simulink model "Pendulum"  (R2013a)
settings: Solver=ode1  SolverMode=SingleTasking  StartTime=0.0  StopTime=inf  FixedStep=0.01  RelTol=1e-3
InitFcn:
  | fuzzycontroller1=readfis('fuzzy1.fis');
  | fuzzycontroller2=readfis('fuzzy2.fis');
  | fuzzypid=readfis('fuzzy3.fis');
libraries: neural x91, fuzblock x9
(part 2 of 2)

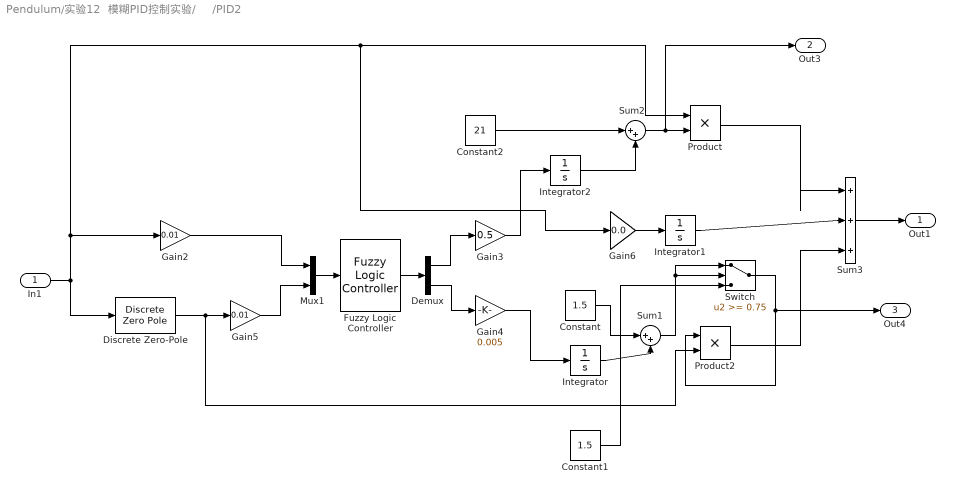
== system Pendulum/实验12  模糊PID控制实验/     /PID2 ==
  In1 : Inport
  Constant : Constant  Value=1.5
  Constant1 : Constant  Value=1.5
  Constant2 : Constant  Value=21
  Demux : Demux  Outputs=2
  Discrete Zero-Pole : DiscreteZeroPole  Poles=[0]  Gain=35  SampleTime=0.01
  Fuzzy Logic Controller : fuzblock/Fuzzy Logic  Controller  fis=fuzzypid
  Gain2 : Gain  Gain=0.01  SaturateOnIntegerOverflow=on  OutDataTypeStr=Inherit: Same as input  ParamDataTypeStr=Inherit: Same as input
  Gain3 : Gain  Gain=0.5  SaturateOnIntegerOverflow=on  OutDataTypeStr=Inherit: Same as input  ParamDataTypeStr=Inherit: Same as input
  Gain4 : Gain  Gain=0.005  SaturateOnIntegerOverflow=on  OutDataTypeStr=Inherit: Same as input  ParamDataTypeStr=Inherit: Same as input
  Gain5 : Gain  Gain=0.01  SaturateOnIntegerOverflow=on  OutDataTypeStr=Inherit: Same as input  ParamDataTypeStr=Inherit: Same as input
  Gain6 : Gain  Gain=0.0  SaturateOnIntegerOverflow=on  OutDataTypeStr=Inherit: Same as input  ParamDataTypeStr=Inherit: Same as input
  Integrator : Integrator
  Integrator1 : Integrator
  Integrator2 : Integrator
  Mux1 : Mux  Inputs=2
  Product : Product  SaturateOnIntegerOverflow=on  OutDataTypeStr=Inherit: Same as first input
  Product2 : Product  SaturateOnIntegerOverflow=on  OutDataTypeStr=Inherit: Same as first input
  Sum1 : Sum  Inputs=|++  SaturateOnIntegerOverflow=on
  Sum2 : Sum  Inputs=|++  SaturateOnIntegerOverflow=on
  Sum3 : Sum  Inputs=|+++  SaturateOnIntegerOverflow=on
  Switch : Switch  Threshold=0.75  SaturateOnIntegerOverflow=on
  Out1 : Outport
  Out3 : Outport  Port=2
  Out4 : Outport  Port=3
  wires:
  Product2/1 -> Sum3/3
  Constant1/1 -> Switch/3
  Sum1/1 -> Switch/2, Switch/1
  Switch/1 -> Out4/1, Product2/1
  Integrator/1 -> Sum1/2
  Sum3/1 -> Out1/1
  Constant/1 -> Sum1/1
  Demux/2 -> Gain4/1
  Gain6/1 -> Integrator1/1
  Product/1 -> Sum3/1
  Gain2/1 -> Mux1/1
  Gain4/1 -> Integrator/1
  Fuzzy Logic Controller/1 -> Demux/1
  Gain5/1 -> Mux1/2
  Demux/1 -> Gain3/1
  Gain3/1 -> Integrator2/1
  Sum2/1 -> Out3/1, Product/2
  Mux1/1 -> Fuzzy Logic Controller/1
  Integrator2/1 -> Sum2/2
  Constant2/1 -> Sum2/1
  Integrator1/1 -> Sum3/2
  Discrete Zero-Pole/1 -> Gain5/1, Product2/2
  In1/1 -> Discrete Zero-Pole/1, Gain2/1, Product/1, Gain6/1

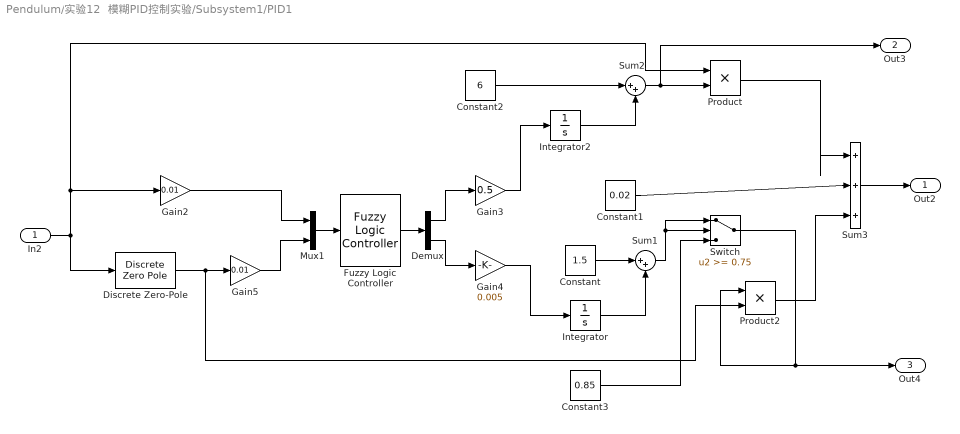
== system Pendulum/实验12  模糊PID控制实验/Subsystem1/PID1 ==
  In2 : Inport
  Constant : Constant  Value=1.5
  Constant1 : Constant  Value=0.02
  Constant2 : Constant  Value=6
  Constant3 : Constant  Value=0.85
  Demux : Demux  Outputs=2
  Discrete Zero-Pole : DiscreteZeroPole  Poles=[0]  Gain=35  SampleTime=0.01
  Fuzzy Logic Controller : fuzblock/Fuzzy Logic  Controller  fis=fuzzypid
  Gain2 : Gain  Gain=0.01  SaturateOnIntegerOverflow=on  OutDataTypeStr=Inherit: Same as input  ParamDataTypeStr=Inherit: Same as input
  Gain3 : Gain  Gain=0.5  SaturateOnIntegerOverflow=on  OutDataTypeStr=Inherit: Same as input  ParamDataTypeStr=Inherit: Same as input
  Gain4 : Gain  Gain=0.005  SaturateOnIntegerOverflow=on  OutDataTypeStr=Inherit: Same as input  ParamDataTypeStr=Inherit: Same as input
  Gain5 : Gain  Gain=0.01  SaturateOnIntegerOverflow=on  OutDataTypeStr=Inherit: Same as input  ParamDataTypeStr=Inherit: Same as input
  Integrator : Integrator
  Integrator2 : Integrator
  Mux1 : Mux  Inputs=2
  Product : Product  SaturateOnIntegerOverflow=on  OutDataTypeStr=Inherit: Same as first input
  Product2 : Product  SaturateOnIntegerOverflow=on  OutDataTypeStr=Inherit: Same as first input
  Sum1 : Sum  Inputs=|++  SaturateOnIntegerOverflow=on
  Sum2 : Sum  Inputs=|++  SaturateOnIntegerOverflow=on
  Sum3 : Sum  Inputs=|+++  SaturateOnIntegerOverflow=on
  Switch : Switch  Threshold=0.75  SaturateOnIntegerOverflow=on
  Out2 : Outport
  Out3 : Outport  Port=2
  Out4 : Outport  Port=3
  wires:
  Sum3/1 -> Out2/1
  Discrete Zero-Pole/1 -> Gain5/1, Product2/2
  Switch/1 -> Out4/1, Product2/1
  Product2/1 -> Sum3/3
  In2/1 -> Discrete Zero-Pole/1, Gain2/1, Product/1
  Constant3/1 -> Switch/3
  Fuzzy Logic Controller/1 -> Demux/1
  Sum2/1 -> Out3/1, Product/2
  Gain5/1 -> Mux1/2
  Constant2/1 -> Sum2/1
  Constant/1 -> Sum1/1
  Mux1/1 -> Fuzzy Logic Controller/1
  Constant1/1 -> Sum3/2
  Integrator/1 -> Sum1/2
  Demux/1 -> Gain3/1
  Demux/2 -> Gain4/1
  Product/1 -> Sum3/1
  Sum1/1 -> Switch/2, Switch/1
  Gain3/1 -> Integrator2/1
  Gain2/1 -> Mux1/1
  Integrator2/1 -> Sum2/2
  Gain4/1 -> Integrator/1

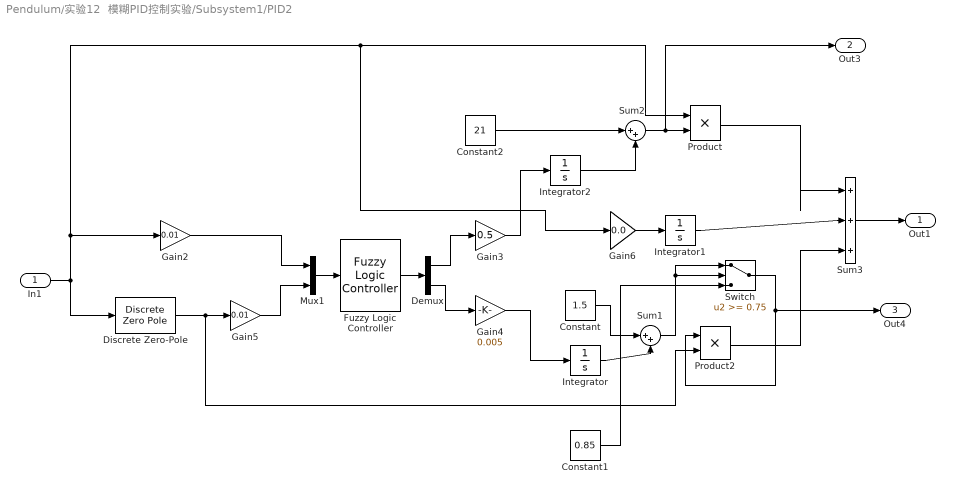
== system Pendulum/实验12  模糊PID控制实验/Subsystem1/PID2 ==
  In1 : Inport
  Constant : Constant  Value=1.5
  Constant1 : Constant  Value=0.85
  Constant2 : Constant  Value=21
  Demux : Demux  Outputs=2
  Discrete Zero-Pole : DiscreteZeroPole  Poles=[0]  Gain=35  SampleTime=0.01
  Fuzzy Logic Controller : fuzblock/Fuzzy Logic  Controller  fis=fuzzypid
  Gain2 : Gain  Gain=0.01  SaturateOnIntegerOverflow=on  OutDataTypeStr=Inherit: Same as input  ParamDataTypeStr=Inherit: Same as input
  Gain3 : Gain  Gain=0.5  SaturateOnIntegerOverflow=on  OutDataTypeStr=Inherit: Same as input  ParamDataTypeStr=Inherit: Same as input
  Gain4 : Gain  Gain=0.005  SaturateOnIntegerOverflow=on  OutDataTypeStr=Inherit: Same as input  ParamDataTypeStr=Inherit: Same as input
  Gain5 : Gain  Gain=0.01  SaturateOnIntegerOverflow=on  OutDataTypeStr=Inherit: Same as input  ParamDataTypeStr=Inherit: Same as input
  Gain6 : Gain  Gain=0.0  SaturateOnIntegerOverflow=on  OutDataTypeStr=Inherit: Same as input  ParamDataTypeStr=Inherit: Same as input
  Integrator : Integrator
  Integrator1 : Integrator
  Integrator2 : Integrator
  Mux1 : Mux  Inputs=2
  Product : Product  SaturateOnIntegerOverflow=on  OutDataTypeStr=Inherit: Same as first input
  Product2 : Product  SaturateOnIntegerOverflow=on  OutDataTypeStr=Inherit: Same as first input
  Sum1 : Sum  Inputs=|++  SaturateOnIntegerOverflow=on
  Sum2 : Sum  Inputs=|++  SaturateOnIntegerOverflow=on
  Sum3 : Sum  Inputs=|+++  SaturateOnIntegerOverflow=on
  Switch : Switch  Threshold=0.75  SaturateOnIntegerOverflow=on
  Out1 : Outport
  Out3 : Outport  Port=2
  Out4 : Outport  Port=3
  wires:
  Product2/1 -> Sum3/3
  Constant1/1 -> Switch/3
  Sum1/1 -> Switch/2, Switch/1
  Switch/1 -> Out4/1, Product2/1
  Integrator/1 -> Sum1/2
  Sum3/1 -> Out1/1
  Constant/1 -> Sum1/1
  Demux/2 -> Gain4/1
  Gain6/1 -> Integrator1/1
  Product/1 -> Sum3/1
  Gain2/1 -> Mux1/1
  Gain4/1 -> Integrator/1
  Fuzzy Logic Controller/1 -> Demux/1
  Gain5/1 -> Mux1/2
  Demux/1 -> Gain3/1
  Gain3/1 -> Integrator2/1
  Sum2/1 -> Out3/1, Product/2
  Mux1/1 -> Fuzzy Logic Controller/1
  Integrator2/1 -> Sum2/2
  Constant2/1 -> Sum2/1
  Integrator1/1 -> Sum3/2
  Discrete Zero-Pole/1 -> Gain5/1, Product2/2
  In1/1 -> Discrete Zero-Pole/1, Gain2/1, Product/1, Gain6/1

== system Pendulum/实验13  神经网络控制实验/神经网络控制器/BP Neural Network ==
  note: 隐层
  note: 输出层
  "p{1}" : Inport  PortDimensions=4
  Layer 1 : Subsystem
  Layer 2 : Subsystem
  "y{1}" : Outport  InitialOutput=0
  wires:
  "p{1}"/1 -> Layer 1/1("p{1}")
  Layer 1/1("a{1}") -> [feedback1]
  [feedback1] -> Layer 2/1("a{1} ")
  Layer 2/1("a{2}") -> "y{1}"/1

== system Pendulum/实验13  神经网络控制实验/神经网络控制器/RBF Neural Network ==
  note: 隐层
  note: 输出层
  "p{1}" : Inport  PortDimensions=4
  Layer 1 : Subsystem
  Layer 2 : Subsystem
  "y{1}" : Outport  InitialOutput=0
  wires:
  "p{1}"/1 -> Layer 1/1("p{1}")
  Layer 1/1("a{1}") -> [feedback1]
  [feedback1] -> Layer 2/1("a{1} ")
  Layer 2/1("a{2}") -> "y{1}"/1

== system Pendulum/实验4  PID控制实验/只对摆杆角度施加控制/PID1 ==
  In1 : Inport
  Discrete Zero-Pole : DiscreteZeroPole  Poles=[0]  Gain=100  SampleTime=0.01
  Gain : Gain  Gain=Kp
  Gain1 : Gain  Gain=Ki
  Gain2 : Gain  Gain=Kd
  Integrator : Integrator  LimitOutput=on  UpperSaturationLimit=0.01  LowerSaturationLimit=-0.01
  Sum : Sum  Inputs=|+++
  Out1 : Outport
  wires:
  Discrete Zero-Pole/1 -> Sum/3
  Gain1/1 -> Integrator/1
  Gain2/1 -> Discrete Zero-Pole/1
  Integrator/1 -> Sum/2
  Gain/1 -> Sum/1
  Sum/1 -> Out1/1
  In1/1 -> Gain2/1, Gain/1, Gain1/1

== system Pendulum/实验4  PID控制实验/对摆杆角度和小车 位置同时施加控制/PID2 ==
  In1 : Inport
  Discrete Zero-Pole : DiscreteZeroPole  Poles=[0]  Gain=100  SampleTime=0.01
  Gain : Gain  Gain=Kp
  Gain1 : Gain  Gain=Ki
  Gain2 : Gain  Gain=Kd
  Integrator : Integrator  LimitOutput=on  UpperSaturationLimit=0.01  LowerSaturationLimit=-0.01
  Sum : Sum  Inputs=|+++
  Out1 : Outport
  wires:
  Discrete Zero-Pole/1 -> Sum/3
  Gain1/1 -> Integrator/1
  Gain2/1 -> Discrete Zero-Pole/1
  Integrator/1 -> Sum/2
  Gain/1 -> Sum/1
  Sum/1 -> Out1/1
  In1/1 -> Gain2/1, Gain/1, Gain1/1

== system Pendulum/实验4  PID控制实验/对摆杆角度和小车 位置同时施加控制/PID3 ==
  In1 : Inport
  Discrete Zero-Pole : DiscreteZeroPole  Poles=[0]  Gain=100  SampleTime=0.01
  Gain : Gain  Gain=Kp
  Gain1 : Gain  Gain=Ki
  Gain2 : Gain  Gain=Kd
  Integrator : Integrator  LimitOutput=on  UpperSaturationLimit=0.01  LowerSaturationLimit=-0.01
  Sum : Sum  Inputs=|+++
  Out1 : Outport
  wires:
  Discrete Zero-Pole/1 -> Sum/3
  Gain1/1 -> Integrator/1
  Gain2/1 -> Discrete Zero-Pole/1
  Integrator/1 -> Sum/2
  Gain/1 -> Sum/1
  Sum/1 -> Out1/1
  In1/1 -> Gain2/1, Gain/1, Gain1/1

== system Pendulum/实验13  神经网络控制实验/神经网络控制器/BP Neural Network/Layer 1 ==
  "p{1}" : Inport  PortDimensions=4
  Delays 1 : Subsystem
      mask Display: disp('TDL')
  "IW{1,1}" : Subsystem
      mask Display: disp('weight')
  "b{1}" : Constant  Value=[-2.6149835398352681;2.2357175048992701;-1.8583595574267076;1.2412188382088436;-0.71456466032423327;0.016058742464604113;-0.094308202124535473;-0.78098051834080862;1.0581145977002466;-1.9595241811893389;2.1672431536686729;2.6034855087406199]
      mask Display: disp('bias')
  netsum : Sum  Inputs=2  SaturateOnIntegerOverflow=on  InputSameDT=on  OutDataTypeStr=Inherit: Same as first input
  tansig : neural/Transfer Functions/tansig
  "a{1}" : Outport  InitialOutput=[0;0;0;0;0;0;0;0;0;0;0;0]
  wires:
  "p{1}"/1 -> Delays 1/1("p{1}")
  Delays 1/1("pd{1,1}") -> "IW{1,1}"/1("pd{1,1}")
  "IW{1,1}"/1("iz{1,1}") -> netsum/1
  "b{1}"/1 -> netsum/2
  netsum/1 -> tansig/1
  tansig/1 -> "a{1}"/1

== system Pendulum/实验13  神经网络控制实验/神经网络控制器/BP Neural Network/Layer 2 ==
  "a{1} " : Inport  PortDimensions=12
  Delays 1 : Subsystem
      mask Display: disp('TDL')
  "LW{2,1}" : Subsystem
      mask Display: disp('weight')
  "b{2}" : Constant  Value=-0.019497373495995372
      mask Display: disp('bias')
  netsum : Sum  Inputs=2  SaturateOnIntegerOverflow=on  InputSameDT=on  OutDataTypeStr=Inherit: Same as first input
  purelin : neural/Transfer Functions/purelin
  "a{2}" : Outport  InitialOutput=0
  wires:
  "a{1} "/1 -> Delays 1/1("p{2}")
  Delays 1/1("pd{2,1}") -> "LW{2,1}"/1("ad{2,1}")
  "LW{2,1}"/1("lz{2,1}") -> netsum/1
  "b{2}"/1 -> netsum/2
  netsum/1 -> purelin/1
  purelin/1 -> "a{2}"/1

== system Pendulum/实验13  神经网络控制实验/神经网络控制器/RBF Neural Network/Layer 1 ==
  "p{1}" : Inport  PortDimensions=4
  Delays 1 : Subsystem
      mask Display: disp('TDL')
  "IW{1,1}" : Subsystem
      mask Display: disp('weight')
  "b{1}" : Constant  Value=[2.7751820371923257;2.7751820371923257;2.7751820371923257;2.7751820371923257;2.7751820371923257;2.7751820371923257;2.7751820371923257;2.7751820371923257;2.7751820371923257;2.7751820371923257;2.7751820371923257;2.7751820371923257;2.7751820371923257;2.7751820371923257;2.7751820371923257;2.7751820371923257;2.7751820371923257;2.7751820371923257;2.7751820371923257;2.7751820371923257;2.7751820371923257;2.7751820371923257;2.7751820371923257;2.7751820371923257;2.7751820371923257;2.7751820371923257;2.7751820371923257;2.7751820371923257;2.7751820371923257;2.7751820371923257;2.7751820371923257;2.7751820371923257;2.7751820371923257;2.7751820371923257;2.7751820371923257;2.7751820371923257;2.7751820371923257;2.7751820371923257;2.7751820371923257;2.7751820371923257;2.7751820371923257;2.7751820371923257;2.7751820371923257;2.7751820371923257;2.7751820371923257;2.7751820371923257;2.7751820371923257;2.7751820371923257;2.7751820371923257;2.7751820371923257;2.7751820371923257;2.7751820371923257;2.7751820371923257;2.7751820371923257;2.7751820371923257;2.7751820371923257;2.7751820371923257;2.7751820371923257;2.7751820371923257;2.7751820371923257;2.7751820371923257;2.7751820371923257;2.7751820371923257;2.7751820371923257;2.7751820371923257;2.7751820371923257;2.7751820371923257;2.7751820371923257;2.7751820371923257;2.7751820371923257;2.7751820371923257;2.7751820371923257;2.7751820371923257]
      mask Display: disp('bias')
  netprod : Product  SaturateOnIntegerOverflow=on  InputSameDT=on  OutDataTypeStr=Inherit: Same as first input
  radbas : neural/Transfer Functions/radbas
  "a{1}" : Outport  InitialOutput=[0;0;0;0;0;0;0;0;0;0;0;0;0;0;0;0;0;0;0;0;0;0;0;0;0;0;0;0;0;0;0;0;0;0;0;0;0;0;0;0;0;0;0;0;0;0;0;0;0;0;0;0;0;0;0;0;0;0;0;0;0;0;0;0;0;0;0;0;0;0;0;0;0]
  wires:
  "p{1}"/1 -> Delays 1/1("p{1}")
  Delays 1/1("pd{1,1}") -> "IW{1,1}"/1("pd{1,1}")
  "IW{1,1}"/1("iz{1,1}") -> netprod/1
  "b{1}"/1 -> netprod/2
  netprod/1 -> radbas/1
  radbas/1 -> "a{1}"/1

== system Pendulum/实验13  神经网络控制实验/神经网络控制器/RBF Neural Network/Layer 2 ==
  "a{1} " : Inport  PortDimensions=73
  Delays 1 : Subsystem
      mask Display: disp('TDL')
  "LW{2,1}" : Subsystem
      mask Display: disp('weight')
  "b{2}" : Constant  Value=-0.33188542288773992
      mask Display: disp('bias')
  netsum : Sum  Inputs=2  SaturateOnIntegerOverflow=on  InputSameDT=on  OutDataTypeStr=Inherit: Same as first input
  purelin : neural/Transfer Functions/purelin
  "a{2}" : Outport  InitialOutput=0
  wires:
  "a{1} "/1 -> Delays 1/1("p{2}")
  Delays 1/1("pd{2,1}") -> "LW{2,1}"/1("ad{2,1}")
  "LW{2,1}"/1("lz{2,1}") -> netsum/1
  "b{2}"/1 -> netsum/2
  netsum/1 -> purelin/1
  purelin/1 -> "a{2}"/1

== system Pendulum/实验13  神经网络控制实验/神经网络控制器/BP Neural Network/Layer 1/Delays 1 ==
  "p{1}" : Inport  PortDimensions=4
  mux : Mux  Inputs=1
  "pd{1,1}" : Outport
  wires:
  "p{1}"/1 -> mux/1
  mux/1 -> "pd{1,1}"/1

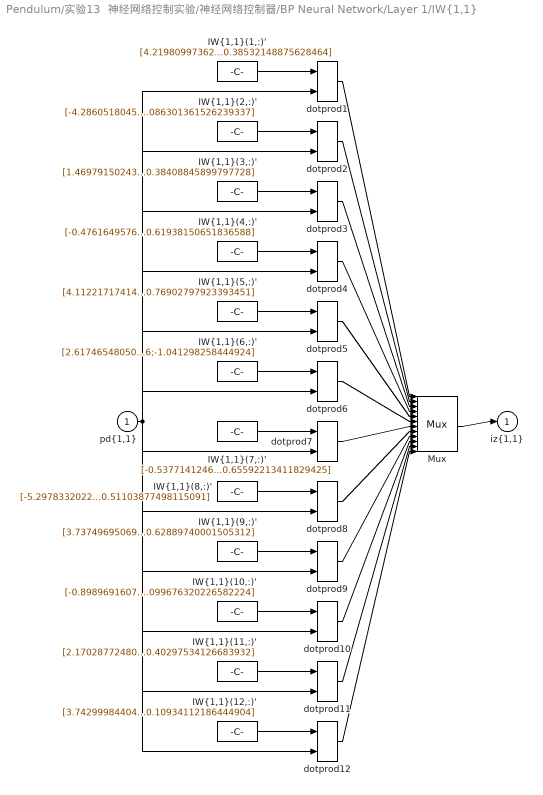
== system Pendulum/实验13  神经网络控制实验/神经网络控制器/BP Neural Network/Layer 1/IW{1,1} ==
  "pd{1,1}" : Inport  PortDimensions=4
  "IW{1,1}(1,:)'" : Constant  Value=[4.2198099736223824;1.3836105378348791;-3.3821166786537664;0.38532148875628464]
      mask Display: disp('weights')
  "IW{1,1}(10,:)'" : Constant  Value=[-0.89896916079005262;-0.83719690218952092;6.9712216279471653;-0.099676320226582224]
      mask Display: disp('weights')
  "IW{1,1}(11,:)'" : Constant  Value=[2.1702877248095773;2.0620343863702146;-0.65349327211843211;0.40297534126683932]
      mask Display: disp('weights')
  "IW{1,1}(12,:)'" : Constant  Value=[3.7429998440421075;-2.1995150028413541;-1.044486577889516;-0.10934112186444904]
      mask Display: disp('weights')
  "IW{1,1}(2,:)'" : Constant  Value=[-4.2860518045013238;1.3298893753918257;-4.7291003819351998;0.086301361526239337]
      mask Display: disp('weights')
  "IW{1,1}(3,:)'" : Constant  Value=[1.4697915024340988;-1.5486100556031892;-4.1075584317347129;-0.38408845899797728]
      mask Display: disp('weights')
  "IW{1,1}(4,:)'" : Constant  Value=[-0.47616495763644751;-1.1066775154194262;3.4697486158917479;0.61938150651836588]
      mask Display: disp('weights')
  "IW{1,1}(5,:)'" : Constant  Value=[4.112217174147208;1.5731852944182383;-2.2298623708405012;0.76902797923393451]
      mask Display: disp('weights')
  "IW{1,1}(6,:)'" : Constant  Value=[2.6174654805091677;1.4887297554514451;-3.3064007623461076;-1.041298258444924]
      mask Display: disp('weights')
  "IW{1,1}(7,:)'" : Constant  Value=[-0.53771412467479052;-0.40827225484336965;-6.8654781754307228;0.65592213411829425]
      mask Display: disp('weights')
  "IW{1,1}(8,:)'" : Constant  Value=[-5.2978332022383192;1.5047659510256346;2.5877056480846519;-0.51103877498115091]
      mask Display: disp('weights')
  "IW{1,1}(9,:)'" : Constant  Value=[3.7374969506989433;-1.789414860758419;-0.56752946895972878;0.62889740001505312]
      mask Display: disp('weights')
  Mux : Mux  Inputs=12
  dotprod{1..12} (12 alike) : neural/Weight Functions/dotprod
  "iz{1,1}" : Outport
  wires:
  "IW{1,1}(1,:)'"/1 -> dotprod1/1
  "pd{1,1}"/1 -> dotprod1/2, dotprod2/2, dotprod3/2, dotprod4/2, dotprod5/2, dotprod6/2, dotprod7/2, dotprod8/2, dotprod9/2, dotprod10/2, dotprod11/2, dotprod12/2
  dotprod1/1 -> Mux/1
  "IW{1,1}(2,:)'"/1 -> dotprod2/1
  dotprod2/1 -> Mux/2
  "IW{1,1}(3,:)'"/1 -> dotprod3/1
  dotprod3/1 -> Mux/3
  "IW{1,1}(4,:)'"/1 -> dotprod4/1
  dotprod4/1 -> Mux/4
  "IW{1,1}(5,:)'"/1 -> dotprod5/1
  dotprod5/1 -> Mux/5
  "IW{1,1}(6,:)'"/1 -> dotprod6/1
  dotprod6/1 -> Mux/6
  "IW{1,1}(7,:)'"/1 -> dotprod7/1
  dotprod7/1 -> Mux/7
  "IW{1,1}(8,:)'"/1 -> dotprod8/1
  dotprod8/1 -> Mux/8
  "IW{1,1}(9,:)'"/1 -> dotprod9/1
  dotprod9/1 -> Mux/9
  "IW{1,1}(10,:)'"/1 -> dotprod10/1
  dotprod10/1 -> Mux/10
  "IW{1,1}(11,:)'"/1 -> dotprod11/1
  dotprod11/1 -> Mux/11
  "IW{1,1}(12,:)'"/1 -> dotprod12/1
  dotprod12/1 -> Mux/12
  Mux/1 -> "iz{1,1}"/1

== system Pendulum/实验13  神经网络控制实验/神经网络控制器/BP Neural Network/Layer 2/Delays 1 ==
  "p{2}" : Inport  PortDimensions=12
  mux : Mux  Inputs=1
  "pd{2,1}" : Outport
  wires:
  "p{2}"/1 -> mux/1
  mux/1 -> "pd{2,1}"/1

== system Pendulum/实验13  神经网络控制实验/神经网络控制器/BP Neural Network/Layer 2/LW{2,1} ==
  "ad{2,1}" : Inport  PortDimensions=12
  "IW{2,1}(1,:)'" : Constant  Value=[-0.36635367987926981;-0.54660331218166769;-0.37003372374556459;-0.22416835299882357;-0.37234015348094707;1.8392819760371051;1.0500227395842805;0.19079880192896481;-0.46017582232306842;0.48070914507964507;0.66483930125499202;0.18163955797980416]
      mask Display: disp('weights')
  Mux : Mux  Inputs=1
  dotprod1 : neural/Weight Functions/dotprod
  "lz{2,1}" : Outport
  wires:
  "IW{2,1}(1,:)'"/1 -> dotprod1/1
  "ad{2,1}"/1 -> dotprod1/2
  dotprod1/1 -> Mux/1
  Mux/1 -> "lz{2,1}"/1

== system Pendulum/实验13  神经网络控制实验/神经网络控制器/RBF Neural Network/Layer 1/Delays 1 ==
  "p{1}" : Inport  PortDimensions=4
  mux : Mux  Inputs=1
  "pd{1,1}" : Outport
  wires:
  "p{1}"/1 -> mux/1
  mux/1 -> "pd{1,1}"/1

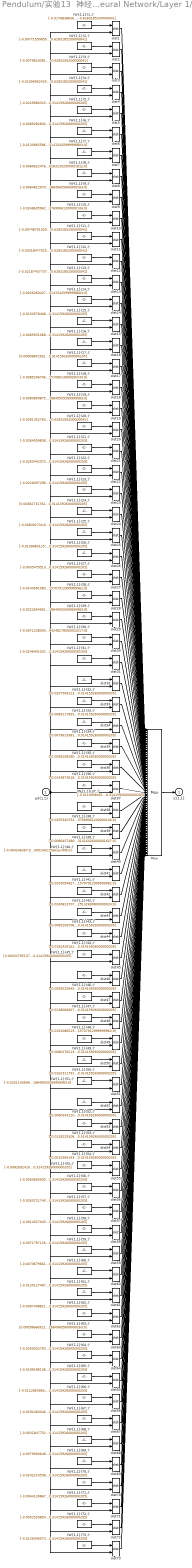
== system Pendulum/实验13  神经网络控制实验/神经网络控制器/RBF Neural Network/Layer 1/IW{1,1} ==
  "pd{1,1}" : Inport  PortDimensions=4
  "IW{1,1}(1,:)'" : Constant  Value=[-0.017683883625000001;-0.067047899999999813;-0.018849505599999983;-0.6283185200000041]
      mask Display: disp('weights')
  "IW{1,1}(10,:)'" : Constant  Value=[-0.024863596250000002;0.067047899999999813;-0.037699061200000106;0]
      mask Display: disp('weights')
  "IW{1,1}(11,:)'" : Constant  Value=[-0.0074870155000000002;0.069841562499999968;0.0062832352000001812;0.6283185200000041]
      mask Display: disp('weights')
  "IW{1,1}(12,:)'" : Constant  Value=[-0.0031847752500000002;0.081016212500000004;0.0094248278000002017;0.6283185200000041]
      mask Display: disp('weights')
  "IW{1,1}(13,:)'" : Constant  Value=[-0.021874377375;0.10336551250000013;-0.021991098200000003;0.6283185200000041]
      mask Display: disp('weights')
  "IW{1,1}(14,:)'" : Constant  Value=[-0.0026260427499999999;0.055873250000000034;-0.0031415425999998803;0]
      mask Display: disp('weights')
  "IW{1,1}(15,:)'" : Constant  Value=[-0.015057840875000001;0.10057185000000007;-0.0094247277999999213;0.31415926000000205]
      mask Display: disp('weights')
  "IW{1,1}(16,:)'" : Constant  Value=[-0.0065651068750000006;0.061460574999999948;-0.012566320399999942;0.31415926000000205]
      mask Display: disp('weights')
  "IW{1,1}(17,:)'" : Constant  Value=[0.00069841562500000008;0.050285925000000009;0.0062832352000001812;0.31415926000000205]
      mask Display: disp('weights')
  "IW{1,1}(18,:)'" : Constant  Value=[-0.0085206706250000007;0.047492262500000056;0.015708013000000243;0]
      mask Display: disp('weights')
  "IW{1,1}(19,:)'" : Constant  Value=[-0.0083809875000000009;0.011174649999999911;-0.018849505599999983;0]
      mask Display: disp('weights')
  "IW{1,1}(2,:)'" : Constant  Value=[-0.0077105085000000002;0.072635225000000025;0.015708013000000243;0.6283185200000041]
      mask Display: disp('weights')
  "IW{1,1}(20,:)'" : Constant  Value=[-0.009135276375000001;-0.086603537500000091;0.0094248278000002017;-0.6283185200000041]
      mask Display: disp('weights')
  "IW{1,1}(21,:)'" : Constant  Value=[-0.026455983875000002;0.002793662499999891;-0.037699061200000106;-0.31415926000000205]
      mask Display: disp('weights')
  "IW{1,1}(22,:)'" : Constant  Value=[-0.026344237375000003;0;-0.028274283400000044;-0.31415926000000205]
      mask Display: disp('weights')
  "IW{1,1}(23,:)'" : Constant  Value=[-0.022600729625;0;-0.025132690800000024;-0.31415926000000205]
      mask Display: disp('weights')
  "IW{1,1}(24,:)'" : Constant  Value=[0.0038273176250000003;0.013968312500000019;0.015708013000000243;0.31415926000000205]
      mask Display: disp('weights')
  "IW{1,1}(25,:)'" : Constant  Value=[-0.008492734;0;-0.015707912999999962;0.31415926000000205]
      mask Display: disp('weights')
  "IW{1,1}(26,:)'" : Constant  Value=[-0.0139683125;0.10895283750000009;-0.0062831351999999008;0.31415926000000205]
      mask Display: disp('weights')
  "IW{1,1}(27,:)'" : Constant  Value=[-0.0035479513749999999;0.030730287500000016;0.018849605600000263;0.31415926000000205]
      mask Display: disp('weights')
  "IW{1,1}(28,:)'" : Constant  Value=[-0.014499108375;-0.011174649999999911;-0.015707912999999962;0]
      mask Display: disp('weights')
  "IW{1,1}(29,:)'" : Constant  Value=[-0.022265490125000002;-0.064254237500000269;-0.018849505599999983;0]
      mask Display: disp('weights')
  "IW{1,1}(3,:)'" : Constant  Value=[-0.0079619381249999999;-0.078222549999999988;0.012566420400000222;-0.6283185200000041]
      mask Display: disp('weights')
  "IW{1,1}(30,:)'" : Constant  Value=[-0.0071238393750000005;0.044698599999999991;0.0094248278000002017;0]
      mask Display: disp('weights')
  "IW{1,1}(31,:)'" : Constant  Value=[-0.02464010325;-0.033523949999999733;-0.021991098200000003;0.31415926000000205]
      mask Display: disp('weights')
  "IW{1,1}(32,:)'" : Constant  Value=[-0.020756912375000002;0.1117464999999998;-0.018849505599999983;0.31415926000000205]
      mask Display: disp('weights')
  "IW{1,1}(33,:)'" : Constant  Value=[-0.008911783375000001;-0.094984525000000111;0.0094248278000002017;-0.31415926000000205]
      mask Display: disp('weights')
  "IW{1,1}(34,:)'" : Constant  Value=[-0.0079619381249999999;0.02514296250000006;0.012566420400000222;-0.31415926000000205]
      mask Display: disp('weights')
  "IW{1,1}(35,:)'" : Constant  Value=[-0.0058108180000000006;-0.058666912500000057;-0.0062831351999999008;-0.31415926000000205]
      mask Display: disp('weights')
  "IW{1,1}(36,:)'" : Constant  Value=[-0.014387361875000001;-0.02514296250000006;-0.015707912999999962;-0.31415926000000205]
      mask Display: disp('weights')
  "IW{1,1}(37,:)'" : Constant  Value=[-0.011090840125000001;0.083809875000000034;0.0062832352000001812;0.31415926000000205]
      mask Display: disp('weights')
  "IW{1,1}(38,:)'" : Constant  Value=[-0.02553407525;0.053079587500000011;-0.037699061200000106;0]
      mask Display: disp('weights')
  "IW{1,1}(39,:)'" : Constant  Value=[-0.0080457480000000001;0.02514296250000006;0.0031416426000001607;0]
      mask Display: disp('weights')
  "IW{1,1}(4,:)'" : Constant  Value=[-0.023969624250000002;0.089397199999999982;-0.031415876000000065;0.6283185200000041]
      mask Display: disp('weights')
  "IW{1,1}(40,:)'" : Constant  Value=[-0.004246367;0.039111275000000036;5.0000000140215661e-008;0]
      mask Display: disp('weights')
  "IW{1,1}(41,:)'" : Constant  Value=[-0.020505482750000002;-0.053079587500000011;-0.015707912999999962;0]
      mask Display: disp('weights')
  "IW{1,1}(42,:)'" : Constant  Value=[-0.024081370750000001;-0.061460575000000031;-0.025132690800000024;0]
      mask Display: disp('weights')
  "IW{1,1}(43,:)'" : Constant  Value=[-0.0085206706250000007;0;-0.018849505599999983;-0.31415926000000205]
      mask Display: disp('weights')
  "IW{1,1}(44,:)'" : Constant  Value=[-0.018242616125;-0.053079587500000011;-0.0094247277999999213;-0.31415926000000205]
      mask Display: disp('weights')
  "IW{1,1}(45,:)'" : Constant  Value=[0.0035479513749999999;0.011174649999999998;0.015708013000000243;-0.31415926000000205]
      mask Display: disp('weights')
  "IW{1,1}(46,:)'" : Constant  Value=[-0.0059225645000000006;0.064254237500000005;-0.0094247277999999213;0.31415926000000205]
      mask Display: disp('weights')
  "IW{1,1}(47,:)'" : Constant  Value=[-0.013800692750000001;0.044698599999999991;5.0000000140215661e-008;-0.31415926000000205]
      mask Display: disp('weights')
  "IW{1,1}(48,:)'" : Constant  Value=[-0.019108651500000001;0.081016212499999962;-0.015707912999999962;0]
      mask Display: disp('weights')
  "IW{1,1}(49,:)'" : Constant  Value=[-0.0080178113749999995;-0.025142962499999887;-0.018849505599999983;-0.31415926000000205]
      mask Display: disp('weights')
  "IW{1,1}(5,:)'" : Constant  Value=[-0.022908032500000002;0.10615917500000002;-0.028274283400000044;0.31415926000000205]
      mask Display: disp('weights')
  "IW{1,1}(50,:)'" : Constant  Value=[-0.016231179125000002;-0.07542888750000018;-0.0062831351999999008;-0.31415926000000205]
      mask Display: disp('weights')
  "IW{1,1}(51,:)'" : Constant  Value=[-0.020114369999999999;-0.041904937499999753;-0.018849505599999983;0]
      mask Display: disp('weights')
  "IW{1,1}(52,:)'" : Constant  Value=[-0.0060343110000000005;0;0.0094248278000002017;-0.31415926000000205]
      mask Display: disp('weights')
  "IW{1,1}(53,:)'" : Constant  Value=[-0.012822910875000001;-0.086603537500000091;-0.0031415425999998803;-0.31415926000000205]
      mask Display: disp('weights')
  "IW{1,1}(54,:)'" : Constant  Value=[-0.0015365143750000001;0;0.0062832352000001812;-0.31415926000000205]
      mask Display: disp('weights')
  "IW{1,1}(55,:)'" : Constant  Value=[-0.0082692410000000001;-0.081016212499999962;0.015708013000000243;-0.31415926000000205]
      mask Display: disp('weights')
  "IW{1,1}(56,:)'" : Constant  Value=[-0.0063695505000000005;0.053079587500000011;0.012566420400000222;0.31415926000000205]
      mask Display: disp('weights')
  "IW{1,1}(57,:)'" : Constant  Value=[-0.026372174000000002;0.002793662499999891;-0.025132690800000024;0.31415926000000205]
      mask Display: disp('weights')
  "IW{1,1}(58,:)'" : Constant  Value=[-0.0014527045000000001;0.058666912500000008;0.0031416426000001607;0.31415926000000205]
      mask Display: disp('weights')
  "IW{1,1}(59,:)'" : Constant  Value=[-0.0071797126250000001;0.047492262500000056;-0.015707912999999962;0.31415926000000205]
      mask Display: disp('weights')
  "IW{1,1}(6,:)'" : Constant  Value=[-0.0069282830000000004;0.097778187500000002;0.0062832352000001812;0.31415926000000205]
      mask Display: disp('weights')
  "IW{1,1}(60,:)'" : Constant  Value=[-0.0070679661250000001;0.064254237500000005;0.018849605600000263;0.31415926000000205]
      mask Display: disp('weights')
  "IW{1,1}(61,:)'" : Constant  Value=[-0.01201274875;-0.069841562499999871;-0.0062831351999999008;-0.31415926000000205]
      mask Display: disp('weights')
  "IW{1,1}(62,:)'" : Constant  Value=[-0.0097498821249999996;0.05028592500000012;5.0000000140215661e-008;0.31415926000000205]
      mask Display: disp('weights')
  "IW{1,1}(63,:)'" : Constant  Value=[0.00058666912499999999;0.061460574999999996;0.018849605600000263;0]
      mask Display: disp('weights')
  "IW{1,1}(64,:)'" : Constant  Value=[-0.025003279375;0.053079587500000011;-0.025132690800000024;0.31415926000000205]
      mask Display: disp('weights')
  "IW{1,1}(65,:)'" : Constant  Value=[-0.019918813625;0.0838098750000002;-0.015707912999999962;0.31415926000000205]
      mask Display: disp('weights')
  "IW{1,1}(66,:)'" : Constant  Value=[-0.0112863965;0.081016212499999962;5.0000000140215661e-008;0.31415926000000205]
      mask Display: disp('weights')
  "IW{1,1}(67,:)'" : Constant  Value=[-0.019248334625000002;-0.002793662500000238;-0.018849505599999983;0.31415926000000205]
      mask Display: disp('weights')
  "IW{1,1}(68,:)'" : Constant  Value=[-0.0031847752500000002;0;0.012566420400000222;0.31415926000000205]
      mask Display: disp('weights')
  "IW{1,1}(69,:)'" : Constant  Value=[-0.0079060648750000004;0.089397199999999982;0.0031416426000001607;0.31415926000000205]
      mask Display: disp('weights')
  "IW{1,1}(7,:)'" : Constant  Value=[-0.012096558625;0.089397199999999982;-0.0031415425999998803;0]
      mask Display: disp('weights')
  "IW{1,1}(70,:)'" : Constant  Value=[-0.024221053875000002;0.078222549999999724;-0.021991098200000003;0.31415926000000205]
      mask Display: disp('weights')
  "IW{1,1}(71,:)'" : Constant  Value=[-0.0044139867500000004;0.083809874999999937;0.012566420400000222;0.31415926000000205]
      mask Display: disp('weights')
  "IW{1,1}(72,:)'" : Constant  Value=[-0.0052520854999999998;0.081016212500000045;0.0094248278000002017;0.31415926000000205]
      mask Display: disp('weights')
  "IW{1,1}(73,:)'" : Constant  Value=[-0.012934657375;0.05028592500000012;-0.0094247277999999213;0.31415926000000205]
      mask Display: disp('weights')
  "IW{1,1}(8,:)'" : Constant  Value=[-0.0060622476250000003;0.086603537500000008;0.0062832352000001812;0]
      mask Display: disp('weights')
  "IW{1,1}(9,:)'" : Constant  Value=[-0.0064812970000000004;0.058666912499999967;0.018849605600000263;0]
      mask Display: disp('weights')
  Mux : Mux  Inputs=73
  dist{1..73} (73 alike) : neural/Weight Functions/dist
  "iz{1,1}" : Outport
  wires:
  "IW{1,1}(1,:)'"/1 -> dist1/1
  "pd{1,1}"/1 -> dist1/2, dist2/2, dist3/2, dist4/2, dist5/2, dist6/2, dist7/2, dist8/2, dist9/2, dist10/2, dist11/2, dist12/2, dist13/2, dist14/2, dist15/2, dist16/2, dist17/2, dist18/2, dist19/2, dist20/2, dist21/2, dist22/2, dist23/2, dist24/2, dist25/2, dist26/2, dist27/2, dist28/2, dist29/2, dist30/2, dist31/2, dist32/2, dist33/2, dist34/2, dist35/2, dist36/2, dist37/2, dist38/2, dist39/2, dist40/2, dist41/2, dist42/2, dist43/2, dist44/2, dist45/2, dist46/2, dist47/2, dist48/2, dist49/2, dist50/2, dist51/2, dist52/2, dist53/2, dist54/2, dist55/2, dist56/2, dist57/2, dist58/2, dist59/2, dist60/2, dist61/2, dist62/2, dist63/2, dist64/2, dist65/2, dist66/2, dist67/2, dist68/2, dist69/2, dist70/2, dist71/2, dist72/2, dist73/2
  dist1/1 -> Mux/1
  "IW{1,1}(2,:)'"/1 -> dist2/1
  dist2/1 -> Mux/2
  "IW{1,1}(3,:)'"/1 -> dist3/1
  dist3/1 -> Mux/3
  "IW{1,1}(4,:)'"/1 -> dist4/1
  dist4/1 -> Mux/4
  "IW{1,1}(5,:)'"/1 -> dist5/1
  dist5/1 -> Mux/5
  "IW{1,1}(6,:)'"/1 -> dist6/1
  dist6/1 -> Mux/6
  "IW{1,1}(7,:)'"/1 -> dist7/1
  dist7/1 -> Mux/7
  "IW{1,1}(8,:)'"/1 -> dist8/1
  dist8/1 -> Mux/8
  "IW{1,1}(9,:)'"/1 -> dist9/1
  dist9/1 -> Mux/9
  "IW{1,1}(10,:)'"/1 -> dist10/1
  dist10/1 -> Mux/10
  "IW{1,1}(11,:)'"/1 -> dist11/1
  dist11/1 -> Mux/11
  "IW{1,1}(12,:)'"/1 -> dist12/1
  dist12/1 -> Mux/12
  "IW{1,1}(13,:)'"/1 -> dist13/1
  dist13/1 -> Mux/13
  "IW{1,1}(14,:)'"/1 -> dist14/1
  dist14/1 -> Mux/14
  "IW{1,1}(15,:)'"/1 -> dist15/1
  dist15/1 -> Mux/15
  "IW{1,1}(16,:)'"/1 -> dist16/1
  dist16/1 -> Mux/16
  "IW{1,1}(17,:)'"/1 -> dist17/1
  dist17/1 -> Mux/17
  "IW{1,1}(18,:)'"/1 -> dist18/1
  dist18/1 -> Mux/18
  "IW{1,1}(19,:)'"/1 -> dist19/1
  dist19/1 -> Mux/19
  "IW{1,1}(20,:)'"/1 -> dist20/1
  dist20/1 -> Mux/20
  "IW{1,1}(21,:)'"/1 -> dist21/1
  dist21/1 -> Mux/21
  "IW{1,1}(22,:)'"/1 -> dist22/1
  dist22/1 -> Mux/22
  "IW{1,1}(23,:)'"/1 -> dist23/1
  dist23/1 -> Mux/23
  "IW{1,1}(24,:)'"/1 -> dist24/1
  dist24/1 -> Mux/24
  "IW{1,1}(25,:)'"/1 -> dist25/1
  dist25/1 -> Mux/25
  "IW{1,1}(26,:)'"/1 -> dist26/1
  dist26/1 -> Mux/26
  "IW{1,1}(27,:)'"/1 -> dist27/1
  dist27/1 -> Mux/27
  "IW{1,1}(28,:)'"/1 -> dist28/1
  dist28/1 -> Mux/28
  "IW{1,1}(29,:)'"/1 -> dist29/1
  dist29/1 -> Mux/29
  "IW{1,1}(30,:)'"/1 -> dist30/1
  dist30/1 -> Mux/30
  "IW{1,1}(31,:)'"/1 -> dist31/1
  dist31/1 -> Mux/31
  "IW{1,1}(32,:)'"/1 -> dist32/1
  dist32/1 -> Mux/32
  "IW{1,1}(33,:)'"/1 -> dist33/1
  dist33/1 -> Mux/33
  "IW{1,1}(34,:)'"/1 -> dist34/1
  dist34/1 -> Mux/34
  "IW{1,1}(35,:)'"/1 -> dist35/1
  dist35/1 -> Mux/35
  "IW{1,1}(36,:)'"/1 -> dist36/1
  dist36/1 -> Mux/36
  "IW{1,1}(37,:)'"/1 -> dist37/1
  dist37/1 -> Mux/37
  "IW{1,1}(38,:)'"/1 -> dist38/1
  dist38/1 -> Mux/38
  "IW{1,1}(39,:)'"/1 -> dist39/1
  dist39/1 -> Mux/39
  "IW{1,1}(40,:)'"/1 -> dist40/1
  dist40/1 -> Mux/40
  "IW{1,1}(41,:)'"/1 -> dist41/1
  dist41/1 -> Mux/41
  "IW{1,1}(42,:)'"/1 -> dist42/1
  dist42/1 -> Mux/42
  "IW{1,1}(43,:)'"/1 -> dist43/1
  dist43/1 -> Mux/43
  "IW{1,1}(44,:)'"/1 -> dist44/1
  dist44/1 -> Mux/44
  "IW{1,1}(45,:)'"/1 -> dist45/1
  dist45/1 -> Mux/45
  "IW{1,1}(46,:)'"/1 -> dist46/1
  dist46/1 -> Mux/46
  "IW{1,1}(47,:)'"/1 -> dist47/1
  dist47/1 -> Mux/47
  "IW{1,1}(48,:)'"/1 -> dist48/1
  dist48/1 -> Mux/48
  "IW{1,1}(49,:)'"/1 -> dist49/1
  dist49/1 -> Mux/49
  "IW{1,1}(50,:)'"/1 -> dist50/1
  dist50/1 -> Mux/50
  "IW{1,1}(51,:)'"/1 -> dist51/1
  dist51/1 -> Mux/51
  "IW{1,1}(52,:)'"/1 -> dist52/1
  dist52/1 -> Mux/52
  "IW{1,1}(53,:)'"/1 -> dist53/1
  dist53/1 -> Mux/53
  "IW{1,1}(54,:)'"/1 -> dist54/1
  dist54/1 -> Mux/54
  "IW{1,1}(55,:)'"/1 -> dist55/1
  dist55/1 -> Mux/55
  "IW{1,1}(56,:)'"/1 -> dist56/1
  dist56/1 -> Mux/56
  "IW{1,1}(57,:)'"/1 -> dist57/1
  dist57/1 -> Mux/57
  "IW{1,1}(58,:)'"/1 -> dist58/1
  dist58/1 -> Mux/58
  "IW{1,1}(59,:)'"/1 -> dist59/1
  dist59/1 -> Mux/59
  "IW{1,1}(60,:)'"/1 -> dist60/1
  dist60/1 -> Mux/60
  "IW{1,1}(61,:)'"/1 -> dist61/1
  dist61/1 -> Mux/61
  "IW{1,1}(62,:)'"/1 -> dist62/1
  dist62/1 -> Mux/62
  "IW{1,1}(63,:)'"/1 -> dist63/1
  dist63/1 -> Mux/63
  "IW{1,1}(64,:)'"/1 -> dist64/1
  dist64/1 -> Mux/64
  "IW{1,1}(65,:)'"/1 -> dist65/1
  dist65/1 -> Mux/65
  "IW{1,1}(66,:)'"/1 -> dist66/1
  dist66/1 -> Mux/66
  "IW{1,1}(67,:)'"/1 -> dist67/1
  dist67/1 -> Mux/67
  "IW{1,1}(68,:)'"/1 -> dist68/1
  dist68/1 -> Mux/68
  "IW{1,1}(69,:)'"/1 -> dist69/1
  dist69/1 -> Mux/69
  "IW{1,1}(70,:)'"/1 -> dist70/1
  dist70/1 -> Mux/70
  "IW{1,1}(71,:)'"/1 -> dist71/1
  dist71/1 -> Mux/71
  "IW{1,1}(72,:)'"/1 -> dist72/1
  dist72/1 -> Mux/72
  "IW{1,1}(73,:)'"/1 -> dist73/1
  dist73/1 -> Mux/73
  Mux/1 -> "iz{1,1}"/1

== system Pendulum/实验13  神经网络控制实验/神经网络控制器/RBF Neural Network/Layer 2/Delays 1 ==
  "p{2}" : Inport  PortDimensions=73
  mux : Mux  Inputs=1
  "pd{2,1}" : Outport
  wires:
  "p{2}"/1 -> mux/1
  mux/1 -> "pd{2,1}"/1

== system Pendulum/实验13  神经网络控制实验/神经网络控制器/RBF Neural Network/Layer 2/LW{2,1} ==
  "ad{2,1}" : Inport  PortDimensions=73
  "IW{2,1}(1,:)'" : Constant  Value=[17.714450398486765;-80.251197008868161;-23.608696586777878;4.0701511228714882;80355.847456389398;-1235958.2748804193;-1612.141592306687;2408.5429108216372;-1196.6763270974204;339.07303160541278;43.046012373513854;36.993458905742386;-4.4993388900842746;-1983.146643718808;-1139725.0217930295;-1249176.6071430705;-369107.51689889934;1146.1197213937871;1984.7241113945588;6.9997180087908397;3517.7329944024373;-16492.582004807067;20796.414728121057;55217.145040673648;-33839.48864957875;723634.07085281494;-57086.735145848739;-8419.7441552749897;6545.0619801268331;-1778.7948570185047;896.3011966498317;-115878.62729931776;-1895.5083498003596;2624.7269317486052;-9516.8679666278222;-23730.064323560815;164361.83967184537;-159.64191868321555;3532.6689577832481;1582.0446565399068;-11012.092208995211;-4817.9120375496768;-9539.9126710704604;23617.834012922023;-5668.2454097549889;1120079.594521787;-583.14104612919766;218.31471882102466;12436.887954478369;-29083.841860562861;13833.734498447169;-9715.2914590473665;13584.601180709338;18661.453784999765;422.79662960021057;401657.38581957656;-27696.724136237292;286513.4245213134;382744.08000633103;-201104.22730462308;10564.450496042566;306821.55604460085;-609.66898202514142;98864.364841482995;894100.29944076471;-722427.85775299987;47604.690631959042;-25858.679789167982;2339327.005271046;-375528.8437356677;1878666.8838316365;-2717531.8948300509;-509922.65965038852]
      mask Display: disp('weights')
  Mux : Mux  Inputs=1
  dotprod1 : neural/Weight Functions/dotprod
  "lz{2,1}" : Outport
  wires:
  "IW{2,1}(1,:)'"/1 -> dotprod1/1
  "ad{2,1}"/1 -> dotprod1/2
  dotprod1/1 -> Mux/1
  Mux/1 -> "lz{2,1}"/1
